simulink model "MINI_Simscape_Assignment_03"  (R2020b)
settings: Solver=FixedStepAuto  StartTime=0.0  StopTime=10  FixedStep=0.001  MaxStep=0.01  RelTol=1e-3
InitFcn:
  | parameters;
model workspace: external: MATLAB File /Users/toricolthurst/School/ECE598IntroToHumanoid/git_humanoid/Project_Matlab/Simulation_DataFile.m (data not in the file)
values from neighbouring files (symbols this model uses):
  Butter_order = 4    [parameters.m]
  Butter_order_IMU = 8    [parameters.m]
undefined symbols (not defined in the file or in its folder): smiData, X, Y, Z
libraries: sm_lib x382, nesl_utility x115, dsparch4 x19, simulink x1
(part 1 of 8)
settings Model: Creator=kggim2  LastModifiedBy=toricolthurst
settings ExplorerConfigSet: InternalSimMechanicsExplorerSettings="<ExplorerConfiguration><canonicalview>default</canonicalview><AnimationSetting><BasePlaybackSpeed>1.0</BasePlaybackSpeed><PlaybackSpeedFactor>1.0</PlaybackSpeedFactor></AnimationSetting><TilePanel><TileInfo><Tiles Columns=\"1\" Count=\"1\" Rows=\"1\"><Column Weight=\"1\"/><Row Weight=\"1\"/><Tile Height=\"1\" Width=\"1\" X=\"0\" Y=\"0\"/></Tiles></TileInfo><SceneInfo><SceneViewer><BGColor><R>0.800000011920928955</R><G>1</G><B>1</B></BGColor><Camera><DoPerspective>off</DoPerspective><Position><X>108.935689512798632</X><Y>53.7617455070637718</Y><Z>50.6647866990595901</Z></Position><Center><X>0.674444181912173146</X><Y>0.341777914819902773</Y><Z>0.208581845546273847</Z></Center><Up><X>-0.338601749819323006</X><Y>-0.185140442280279371</Y><Z>0.922535566605187762</Z></Up><ViewLimDist>1</ViewLimDist><YLim>0.289357950952195409</YLim><XLim>0.308353002437022183</XLim></Camera></SceneViewer></SceneInfo></TilePanel><MechEditorPanel><Cameras/><GfxPanelCameraMap/><VideoCreator><PlaybackSpeedRatio>1.0</PlaybackSpeedRatio><FrameRate>30</FrameRate><VideoFormat>MPEG-4</VideoFormat><FrameSize>auto</FrameSize></VideoCreator></MechEditorPanel></ExplorerConfiguration>"

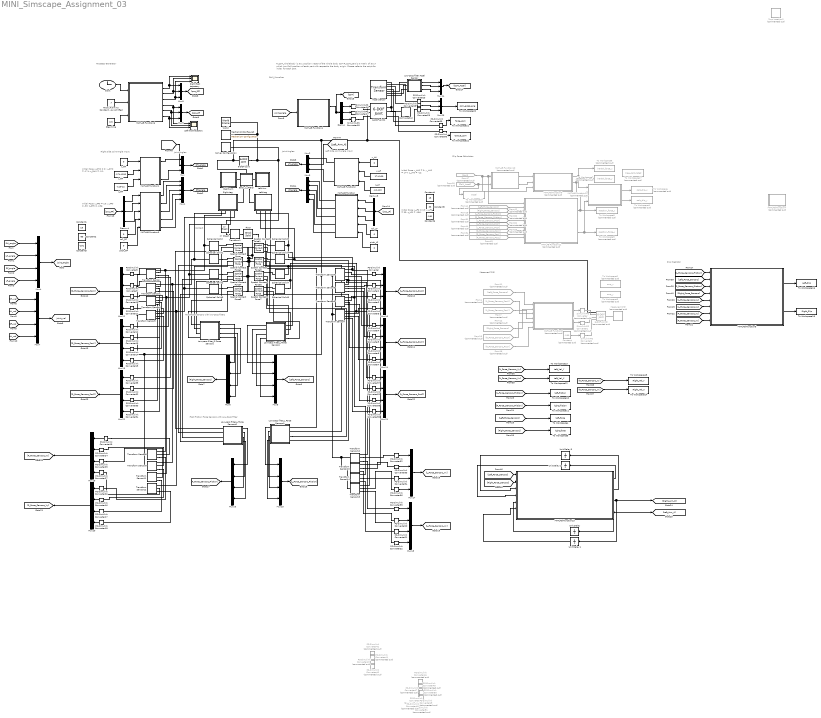
== system MINI_Simscape_Assignment_03 ==
  note: Slip Predictor
  note: P_CoM_wholebody is 3x1 position vector of the whole body CoM
      | P_CoM_part is a matrix of 3x17 which is a CoM position of each part with respect to the body origin. Please refer to the script for index for each part.
  note: Foot Force sensors with low-pass filters
  note: Footstep Generator
  note: CoM_Visualize
  note: Joint Angles
  note: Right Side Joint Angle Input
  note: Left Side Joint Angle Input
  note: Contact
  note: Joint Angles
  note: Initial Pose
      | x_RH0 = 0;
      | y_RH0 = -174;
      | z_RH0 = -12;
  note: Initial Pose
      | x_RF0 = 15;
      | y_RF0 = -33;
      | z_RF0 = -196;
  note: Initial Pose
      | x_LF0 = 15;
      | y_LF0 = 33;
      | z_LF0 = -196;
  note: Initial Pose
      | x_LH0 = 0;
      | y_LH0 = 174;
      | z_LH0 = -12;
  note: Measured ZMP
  note: Slip Force Calculator
  note: Foot Friction Force Sensors with Low-Pass Filter
  6-DOF Joint : sm_lib/Joints/6-DOF Joint  JointMode=Normal  SenseConstraintForce=off  SenseConstraintForceX=off  SenseConstraintForceY=off  SenseConstraintForceZ=off  SenseConstraintTorque=off  SenseConstraintTorqueX=off  SenseConstraintTorqueY=off  SenseConstraintTorqueZ=off  SenseTotalForce=off  SenseTotalForceX=off  SenseTotalForceY=off  SenseTotalForceZ=off  SenseTotalTorque=off  SenseTotalTorqueX=off  SenseTotalTorqueY=off  SenseTotalTorqueZ=off  CompositeWrenchDir=FollowerOnBase  CompositeWrenchFrame=BaseFrame  PxEquilibriumPosition=0  PxEquilibriumPositionUnits=m  PxSpringStiffness=0  PxSpringStiffnessUnits=N/m  PxDampingCoefficient=0  PxDampingCoefficientUnits=N/(m/s)  PxTorqueActuationMode=NoTorque  PxMotionActuationMode=ComputedMotion  PxSensePosition=off  PxSenseVelocity=off  PxSenseAcceleration=off  PxSenseTorqueForce=off  PxSenseLowerLimitTorqueForce=off  PxSenseUpperLimitTorqueForce=off  PxLowerLimitSpecify=off  PxLowerLimitBound=-1  PxLowerLimitBoundUnits=m  PxLowerLimitStiffness=1e6  PxLowerLimitStiffnessUnits=N/m  PxLowerLimitDamping=1e3  PxLowerLimitDampingUnits=N/(m/s)  PxLowerLimitTransitionRegionWidth=1e-4  PxLowerLimitTransitionRegionWidthUnits=m  PxUpperLimitSpecify=off  PxUpperLimitBound=1  PxUpperLimitBoundUnits=m  PxUpperLimitStiffness=1e6  PxUpperLimitStiffnessUnits=N/m  PxUpperLimitDamping=1e3  PxUpperLimitDampingUnits=N/(m/s)  PxUpperLimitTransitionRegionWidth=1e-4  PxUpperLimitTransitionRegionWidthUnits=m  PxPositionTargetSpecify=off  PxPositionTargetPriority=High  PxPositionTargetValue=0  PxPositionTargetValueUnits=m  PxVelocityTargetSpecify=off  PxVelocityTargetPriority=High  PxVelocityTargetValue=0  PxVelocityTargetValueUnits=m/s  PyEquilibriumPosition=0  PyEquilibriumPositionUnits=m  PySpringStiffness=0  PySpringStiffnessUnits=N/m  PyDampingCoefficient=0  PyDampingCoefficientUnits=N/(m/s)  PyTorqueActuationMode=NoTorque  PyMotionActuationMode=ComputedMotion  PySensePosition=off  PySenseVelocity=off  PySenseAcceleration=off  PySenseTorqueForce=off  PySenseLowerLimitTorqueForce=off  PySenseUpperLimitTorqueForce=off  PyLowerLimitSpecify=off  PyLowerLimitBound=-1  PyLowerLimitBoundUnits=m  PyLowerLimitStiffness=1e6  PyLowerLimitStiffnessUnits=N/m  PyLowerLimitDamping=1e3  PyLowerLimitDampingUnits=N/(m/s)  PyLowerLimitTransitionRegionWidth=1e-4  PyLowerLimitTransitionRegionWidthUnits=m  PyUpperLimitSpecify=off  PyUpperLimitBound=1  PyUpperLimitBoundUnits=m  PyUpperLimitStiffness=1e6  PyUpperLimitStiffnessUnits=N/m  PyUpperLimitDamping=1e3  PyUpperLimitDampingUnits=N/(m/s)  PyUpperLimitTransitionRegionWidth=1e-4  PyUpperLimitTransitionRegionWidthUnits=m  PyPositionTargetSpecify=off  PyPositionTargetPriority=High  PyPositionTargetValue=0  PyPositionTargetValueUnits=m  PyVelocityTargetSpecify=off  PyVelocityTargetPriority=High  PyVelocityTargetValue=0  PyVelocityTargetValueUnits=m/s  PzEquilibriumPosition=0  PzEquilibriumPositionUnits=m  PzSpringStiffness=0  PzSpringStiffnessUnits=N/m  PzDampingCoefficient=0  PzDampingCoefficientUnits=N/(m/s)  PzTorqueActuationMode=NoTorque  PzMotionActuationMode=ComputedMotion  PzSensePosition=off  PzSenseVelocity=off  PzSenseAcceleration=off  PzSenseTorqueForce=off  PzSenseLowerLimitTorqueForce=off  PzSenseUpperLimitTorqueForce=off  PzLowerLimitSpecify=off  PzLowerLimitBound=-1  PzLowerLimitBoundUnits=m  PzLowerLimitStiffness=1e6  PzLowerLimitStiffnessUnits=N/m  PzLowerLimitDamping=1e3  PzLowerLimitDampingUnits=N/(m/s)  PzLowerLimitTransitionRegionWidth=1e-4  PzLowerLimitTransitionRegionWidthUnits=m  PzUpperLimitSpecify=off  PzUpperLimitBound=1  PzUpperLimitBoundUnits=m  PzUpperLimitStiffness=1e6  PzUpperLimitStiffnessUnits=N/m  PzUpperLimitDamping=1e3  PzUpperLimitDampingUnits=N/(m/s)  PzUpperLimitTransitionRegionWidth=1e-4  PzUpperLimitTransitionRegionWidthUnits=m  PzPositionTargetSpecify=off  PzPositionTargetPriority=High  PzPositionTargetValue=0  PzPositionTargetValueUnits=m  PzVelocityTargetSpecify=off  PzVelocityTargetPriority=High  PzVelocityTargetValue=0  PzVelocityTargetValueUnits=m/s  SphDefPosRotationMethod=None  SphDefPosRotationAngleUnits=deg  SphDefPosRotationStandardAxis=+Z  SphDefPosRotationAngle=0.0  SphDefPosRotationArbitraryAxis=[0 0 1]  SphDefPosFollAlignAxisA=+X  SphDefPosBaseAlignAxisA=+Y  SphDefPosFollAlignAxisB=+Y  SphDefPosBaseAlignAxisB=+Z  SphDefPosRotationSequenceAxes=FollowerAxes  SphDefPosRotationSequence=XYX  SphDefPosRotationSequenceAngles=[0 0 0]  SphDefPosRotationSequenceAnglesUnits=deg  SphDefPosRotationMatrix=[1 0 0; 0 1 0; 0 0 1]  SphEqPosRotationMethod=None  SphEqPosRotationAngleUnits=deg  SphEqPosRotationStandardAxis=+Z  SphEqPosRotationAngle=0.0  SphEqPosRotationArbitraryAxis=[0 0 1]  SphEqPosFollAlignAxisA=+X  SphEqPosBaseAlignAxisA=+Y  SphEqPosFollAlignAxisB=+Y  SphEqPosBaseAlignAxisB=+Z  SphEqPosRotationSequenceAxes=FollowerAxes  SphEqPosRotationSequence=XYX  SphEqPosRotationSequenceAngles=[0 0 0]  SphEqPosRotationSequenceAnglesUnits=deg  SphEqPosRotationMatrix=[1 0 0; 0 1 0; 0 0 1]  SphSpringStiffness=0  SphSpringStiffnessUnits=N*m/deg  SphDampingCoefficient=0  SphDampingCoefficientUnits=N*m/(deg/s)  SphActuateTorqueX=off  SphActuateTorqueY=off  SphActuateTorqueZ=off  SphActuateTorque=off  SphTorqueActuationMode=NoTorque  SphMotionActuationMode=ComputedMotion  SphActuationFrame=BaseFrame  SphSensePosition=off  SphSenseVelocityX=off  SphSenseVelocityY=off  SphSenseVelocityZ=off  SphSenseVelocity=off  SphSenseAccelerationX=off  SphSenseAccelerationY=off  SphSenseAccelerationZ=off  SphSenseAcceleration=off  SphSenseTorqueX=off  SphSenseTorqueY=off  SphSenseTorqueZ=off  SphSenseTorqueForce=off  SphSenseLowerLimitTorqueMag=off  SphSenseUpperLimitTorqueMag=off  SphSensingFrame=BaseFrame  SphLowerLimitSpecify=off  SphLowerLimitBound=15  SphLowerLimitBoundUnits=deg  SphLowerLimitStiffness=1e4  SphLowerLimitStiffnessUnits=N*m/deg  SphLowerLimitDamping=10  SphLowerLimitDampingUnits=N*m/(deg/s)  SphLowerLimitTransitionRegionWidth=0.1  SphLowerLimitTransitionRegionWidthUnits=deg  SphUpperLimitSpecify=off  SphUpperLimitBound=45  SphUpperLimitBoundUnits=deg  SphUpperLimitStiffness=1e4  SphUpperLimitStiffnessUnits=N*m/deg  SphUpperLimitDamping=10  SphUpperLimitDampingUnits=N*m/(deg/s)  SphUpperLimitTransitionRegionWidth=0.1  SphUpperLimitTransitionRegionWidthUnits=deg  SphPositionTargetRotationMethod=None  SphPositionTargetRotationAngleUnits=deg  SphPositionTargetRotationStandardAxis=+Z  SphPositionTargetRotationAngle=0.0  SphPositionTargetRotationArbitraryAxis=[0 0 1]  SphPositionTargetFollAlignAxisA=+X  SphPositionTargetBaseAlignAxisA=+Y  SphPositionTargetFollAlignAxisB=+Y  SphPositionTargetBaseAlignAxisB=+Z  SphPositionTargetRotationSequenceAxes=FollowerAxes  SphPositionTargetRotationSequence=XYX  SphPositionTargetRotationSequenceAngles=[0 0 0]  SphPositionTargetRotationSequenceAnglesUnits=deg  SphPositionTargetRotationMatrix=[1 0 0; 0 1 0; 0 0 1]  SphPositionTargetSpecify=off  SphPositionTargetPriority=High  SphVelocityTargetValue=[0 0 0]  SphVelocityTargetValueUnits=deg/s  SphVelocityTargetSpecify=off  SphVelocityTargetPriority=High  SphVelocityTargetInFollowerFrame=on
  6-DOF Joint1 : sm_lib/Joints/6-DOF Joint  JointMode=Normal  SenseConstraintForce=off  SenseConstraintForceX=off  SenseConstraintForceY=off  SenseConstraintForceZ=off  SenseConstraintTorque=off  SenseConstraintTorqueX=off  SenseConstraintTorqueY=off  SenseConstraintTorqueZ=off  SenseTotalForce=on  SenseTotalForceX=off  SenseTotalForceY=off  SenseTotalForceZ=off  SenseTotalTorque=on  SenseTotalTorqueX=off  SenseTotalTorqueY=off  SenseTotalTorqueZ=off  CompositeWrenchDir=FollowerOnBase  CompositeWrenchFrame=BaseFrame  PxEquilibriumPosition=0  PxEquilibriumPositionUnits=m  PxSpringStiffness=0  PxSpringStiffnessUnits=N/m  PxDampingCoefficient=0  PxDampingCoefficientUnits=N/(m/s)  PxTorqueActuationMode=ComputedTorque  PxMotionActuationMode=InputMotion  PxSensePosition=off  PxSenseVelocity=off  PxSenseAcceleration=off  PxSenseTorqueForce=off  PxSenseLowerLimitTorqueForce=off  PxSenseUpperLimitTorqueForce=off  PxLowerLimitSpecify=off  PxLowerLimitBound=-1  PxLowerLimitBoundUnits=m  PxLowerLimitStiffness=1e6  PxLowerLimitStiffnessUnits=N/m  PxLowerLimitDamping=1e3  PxLowerLimitDampingUnits=N/(m/s)  PxLowerLimitTransitionRegionWidth=1e-4  PxLowerLimitTransitionRegionWidthUnits=m  PxUpperLimitSpecify=off  PxUpperLimitBound=1  PxUpperLimitBoundUnits=m  PxUpperLimitStiffness=1e6  PxUpperLimitStiffnessUnits=N/m  PxUpperLimitDamping=1e3  PxUpperLimitDampingUnits=N/(m/s)  PxUpperLimitTransitionRegionWidth=1e-4  PxUpperLimitTransitionRegionWidthUnits=m  PxPositionTargetSpecify=off  PxPositionTargetPriority=High  PxPositionTargetValue=0  PxPositionTargetValueUnits=m  PxVelocityTargetSpecify=off  PxVelocityTargetPriority=High  PxVelocityTargetValue=0  PxVelocityTargetValueUnits=m/s  PyEquilibriumPosition=0  PyEquilibriumPositionUnits=m  PySpringStiffness=0  PySpringStiffnessUnits=N/m  PyDampingCoefficient=0  PyDampingCoefficientUnits=N/(m/s)  PyTorqueActuationMode=ComputedTorque  PyMotionActuationMode=InputMotion  PySensePosition=off  PySenseVelocity=off  PySenseAcceleration=off  PySenseTorqueForce=off  PySenseLowerLimitTorqueForce=off  PySenseUpperLimitTorqueForce=off  PyLowerLimitSpecify=off  PyLowerLimitBound=-1  PyLowerLimitBoundUnits=m  PyLowerLimitStiffness=1e6  PyLowerLimitStiffnessUnits=N/m  PyLowerLimitDamping=1e3  PyLowerLimitDampingUnits=N/(m/s)  PyLowerLimitTransitionRegionWidth=1e-4  PyLowerLimitTransitionRegionWidthUnits=m  PyUpperLimitSpecify=off  PyUpperLimitBound=1  PyUpperLimitBoundUnits=m  PyUpperLimitStiffness=1e6  PyUpperLimitStiffnessUnits=N/m  PyUpperLimitDamping=1e3  PyUpperLimitDampingUnits=N/(m/s)  PyUpperLimitTransitionRegionWidth=1e-4  PyUpperLimitTransitionRegionWidthUnits=m  PyPositionTargetSpecify=off  PyPositionTargetPriority=High  PyPositionTargetValue=0  PyPositionTargetValueUnits=m  PyVelocityTargetSpecify=off  PyVelocityTargetPriority=High  PyVelocityTargetValue=0  PyVelocityTargetValueUnits=m/s  PzEquilibriumPosition=0  PzEquilibriumPositionUnits=m  PzSpringStiffness=0  PzSpringStiffnessUnits=N/m  PzDampingCoefficient=0  PzDampingCoefficientUnits=N/(m/s)  PzTorqueActuationMode=ComputedTorque  PzMotionActuationMode=InputMotion  PzSensePosition=off  PzSenseVelocity=off  PzSenseAcceleration=off  PzSenseTorqueForce=off  PzSenseLowerLimitTorqueForce=off  PzSenseUpperLimitTorqueForce=off  PzLowerLimitSpecify=off  PzLowerLimitBound=-1  PzLowerLimitBoundUnits=m  PzLowerLimitStiffness=1e6  PzLowerLimitStiffnessUnits=N/m  PzLowerLimitDamping=1e3  PzLowerLimitDampingUnits=N/(m/s)  PzLowerLimitTransitionRegionWidth=1e-4  PzLowerLimitTransitionRegionWidthUnits=m  PzUpperLimitSpecify=off  PzUpperLimitBound=1  PzUpperLimitBoundUnits=m  PzUpperLimitStiffness=1e6  PzUpperLimitStiffnessUnits=N/m  PzUpperLimitDamping=1e3  PzUpperLimitDampingUnits=N/(m/s)  PzUpperLimitTransitionRegionWidth=1e-4  PzUpperLimitTransitionRegionWidthUnits=m  PzPositionTargetSpecify=off  PzPositionTargetPriority=High  PzPositionTargetValue=0  PzPositionTargetValueUnits=m  PzVelocityTargetSpecify=off  PzVelocityTargetPriority=High  PzVelocityTargetValue=0  PzVelocityTargetValueUnits=m/s  SphDefPosRotationMethod=None  SphDefPosRotationAngleUnits=deg  SphDefPosRotationStandardAxis=+Z  SphDefPosRotationAngle=0.0  SphDefPosRotationArbitraryAxis=[0 0 1]  SphDefPosFollAlignAxisA=+X  SphDefPosBaseAlignAxisA=+Y  SphDefPosFollAlignAxisB=+Y  SphDefPosBaseAlignAxisB=+Z  SphDefPosRotationSequenceAxes=FollowerAxes  SphDefPosRotationSequence=XYX  SphDefPosRotationSequenceAngles=[0 0 0]  SphDefPosRotationSequenceAnglesUnits=deg  SphDefPosRotationMatrix=[1 0 0; 0 1 0; 0 0 1]  SphEqPosRotationMethod=None  SphEqPosRotationAngleUnits=deg  SphEqPosRotationStandardAxis=+Z  SphEqPosRotationAngle=0.0  SphEqPosRotationArbitraryAxis=[0 0 1]  SphEqPosFollAlignAxisA=+X  SphEqPosBaseAlignAxisA=+Y  SphEqPosFollAlignAxisB=+Y  SphEqPosBaseAlignAxisB=+Z  SphEqPosRotationSequenceAxes=FollowerAxes  SphEqPosRotationSequence=XYX  SphEqPosRotationSequenceAngles=[0 0 0]  SphEqPosRotationSequenceAnglesUnits=deg  SphEqPosRotationMatrix=[1 0 0; 0 1 0; 0 0 1]  SphSpringStiffness=0  SphSpringStiffnessUnits=N*m/deg  SphDampingCoefficient=0  SphDampingCoefficientUnits=N*m/(deg/s)  SphActuateTorqueX=off  SphActuateTorqueY=off  SphActuateTorqueZ=off  SphActuateTorque=off  SphTorqueActuationMode=NoTorque  SphMotionActuationMode=ComputedMotion  SphActuationFrame=BaseFrame  SphSensePosition=off  SphSenseVelocityX=off  SphSenseVelocityY=off  SphSenseVelocityZ=off  SphSenseVelocity=off  SphSenseAccelerationX=off  SphSenseAccelerationY=off  SphSenseAccelerationZ=off  SphSenseAcceleration=off  SphSenseTorqueX=off  SphSenseTorqueY=off  SphSenseTorqueZ=off  SphSenseTorqueForce=off  SphSenseLowerLimitTorqueMag=off  SphSenseUpperLimitTorqueMag=off  SphSensingFrame=BaseFrame  SphLowerLimitSpecify=off  SphLowerLimitBound=15  SphLowerLimitBoundUnits=deg  SphLowerLimitStiffness=1e4  SphLowerLimitStiffnessUnits=N*m/deg  SphLowerLimitDamping=10  SphLowerLimitDampingUnits=N*m/(deg/s)  SphLowerLimitTransitionRegionWidth=0.1  SphLowerLimitTransitionRegionWidthUnits=deg  SphUpperLimitSpecify=off  SphUpperLimitBound=45  SphUpperLimitBoundUnits=deg  SphUpperLimitStiffness=1e4  SphUpperLimitStiffnessUnits=N*m/deg  SphUpperLimitDamping=10  SphUpperLimitDampingUnits=N*m/(deg/s)  SphUpperLimitTransitionRegionWidth=0.1  SphUpperLimitTransitionRegionWidthUnits=deg  SphPositionTargetRotationMethod=None  SphPositionTargetRotationAngleUnits=deg  SphPositionTargetRotationStandardAxis=+Z  SphPositionTargetRotationAngle=0.0  SphPositionTargetRotationArbitraryAxis=[0 0 1]  SphPositionTargetFollAlignAxisA=+X  SphPositionTargetBaseAlignAxisA=+Y  SphPositionTargetFollAlignAxisB=+Y  SphPositionTargetBaseAlignAxisB=+Z  SphPositionTargetRotationSequenceAxes=FollowerAxes  SphPositionTargetRotationSequence=XYX  SphPositionTargetRotationSequenceAngles=[0 0 0]  SphPositionTargetRotationSequenceAnglesUnits=deg  SphPositionTargetRotationMatrix=[1 0 0; 0 1 0; 0 0 1]  SphPositionTargetSpecify=off  SphPositionTargetPriority=High  SphVelocityTargetValue=[0 0 0]  SphVelocityTargetValueUnits=deg/s  SphVelocityTargetSpecify=off  SphVelocityTargetPriority=High  SphVelocityTargetInFollowerFrame=on
  6-DOF Joint2 : sm_lib/Joints/6-DOF Joint  Commented=on  JointMode=Normal  SenseConstraintForce=off  SenseConstraintForceX=off  SenseConstraintForceY=off  SenseConstraintForceZ=off  SenseConstraintTorque=off  SenseConstraintTorqueX=off  SenseConstraintTorqueY=off  SenseConstraintTorqueZ=off  SenseTotalForce=off  SenseTotalForceX=off  SenseTotalForceY=off  SenseTotalForceZ=off  SenseTotalTorque=off  SenseTotalTorqueX=off  SenseTotalTorqueY=off  SenseTotalTorqueZ=off  CompositeWrenchDir=FollowerOnBase  CompositeWrenchFrame=BaseFrame  PxEquilibriumPosition=0  PxEquilibriumPositionUnits=m  PxSpringStiffness=0  PxSpringStiffnessUnits=N/m  PxDampingCoefficient=0  PxDampingCoefficientUnits=N/(m/s)  PxTorqueActuationMode=ComputedTorque  PxMotionActuationMode=InputMotion  PxSensePosition=off  PxSenseVelocity=off  PxSenseAcceleration=off  PxSenseTorqueForce=off  PxSenseLowerLimitTorqueForce=off  PxSenseUpperLimitTorqueForce=off  PxLowerLimitSpecify=off  PxLowerLimitBound=-1  PxLowerLimitBoundUnits=m  PxLowerLimitStiffness=1e6  PxLowerLimitStiffnessUnits=N/m  PxLowerLimitDamping=1e3  PxLowerLimitDampingUnits=N/(m/s)  PxLowerLimitTransitionRegionWidth=1e-4  PxLowerLimitTransitionRegionWidthUnits=m  PxUpperLimitSpecify=off  PxUpperLimitBound=1  PxUpperLimitBoundUnits=m  PxUpperLimitStiffness=1e6  PxUpperLimitStiffnessUnits=N/m  PxUpperLimitDamping=1e3  PxUpperLimitDampingUnits=N/(m/s)  PxUpperLimitTransitionRegionWidth=1e-4  PxUpperLimitTransitionRegionWidthUnits=m  PxPositionTargetSpecify=off  PxPositionTargetPriority=High  PxPositionTargetValue=0  PxPositionTargetValueUnits=m  PxVelocityTargetSpecify=off  PxVelocityTargetPriority=High  PxVelocityTargetValue=0  PxVelocityTargetValueUnits=m/s  PyEquilibriumPosition=0  PyEquilibriumPositionUnits=m  PySpringStiffness=0  PySpringStiffnessUnits=N/m  PyDampingCoefficient=0  PyDampingCoefficientUnits=N/(m/s)  PyTorqueActuationMode=ComputedTorque  PyMotionActuationMode=InputMotion  PySensePosition=off  PySenseVelocity=off  PySenseAcceleration=off  PySenseTorqueForce=off  PySenseLowerLimitTorqueForce=off  PySenseUpperLimitTorqueForce=off  PyLowerLimitSpecify=off  PyLowerLimitBound=-1  PyLowerLimitBoundUnits=m  PyLowerLimitStiffness=1e6  PyLowerLimitStiffnessUnits=N/m  PyLowerLimitDamping=1e3  PyLowerLimitDampingUnits=N/(m/s)  PyLowerLimitTransitionRegionWidth=1e-4  PyLowerLimitTransitionRegionWidthUnits=m  PyUpperLimitSpecify=off  PyUpperLimitBound=1  PyUpperLimitBoundUnits=m  PyUpperLimitStiffness=1e6  PyUpperLimitStiffnessUnits=N/m  PyUpperLimitDamping=1e3  PyUpperLimitDampingUnits=N/(m/s)  PyUpperLimitTransitionRegionWidth=1e-4  PyUpperLimitTransitionRegionWidthUnits=m  PyPositionTargetSpecify=off  PyPositionTargetPriority=High  PyPositionTargetValue=0  PyPositionTargetValueUnits=m  PyVelocityTargetSpecify=off  PyVelocityTargetPriority=High  PyVelocityTargetValue=0  PyVelocityTargetValueUnits=m/s  PzEquilibriumPosition=0  PzEquilibriumPositionUnits=m  PzSpringStiffness=0  PzSpringStiffnessUnits=N/m  PzDampingCoefficient=0  PzDampingCoefficientUnits=N/(m/s)  PzTorqueActuationMode=ComputedTorque  PzMotionActuationMode=InputMotion  PzSensePosition=off  PzSenseVelocity=off  PzSenseAcceleration=off  PzSenseTorqueForce=off  PzSenseLowerLimitTorqueForce=off  PzSenseUpperLimitTorqueForce=off  PzLowerLimitSpecify=off  PzLowerLimitBound=-1  PzLowerLimitBoundUnits=m  PzLowerLimitStiffness=1e6  PzLowerLimitStiffnessUnits=N/m  PzLowerLimitDamping=1e3  PzLowerLimitDampingUnits=N/(m/s)  PzLowerLimitTransitionRegionWidth=1e-4  PzLowerLimitTransitionRegionWidthUnits=m  PzUpperLimitSpecify=off  PzUpperLimitBound=1  PzUpperLimitBoundUnits=m  PzUpperLimitStiffness=1e6  PzUpperLimitStiffnessUnits=N/m  PzUpperLimitDamping=1e3  PzUpperLimitDampingUnits=N/(m/s)  PzUpperLimitTransitionRegionWidth=1e-4  PzUpperLimitTransitionRegionWidthUnits=m  PzPositionTargetSpecify=off  PzPositionTargetPriority=High  PzPositionTargetValue=0  PzPositionTargetValueUnits=m  PzVelocityTargetSpecify=off  PzVelocityTargetPriority=High  PzVelocityTargetValue=0  PzVelocityTargetValueUnits=m/s  SphDefPosRotationMethod=None  SphDefPosRotationAngleUnits=deg  SphDefPosRotationStandardAxis=+Z  SphDefPosRotationAngle=0.0  SphDefPosRotationArbitraryAxis=[0 0 1]  SphDefPosFollAlignAxisA=+X  SphDefPosBaseAlignAxisA=+Y  SphDefPosFollAlignAxisB=+Y  SphDefPosBaseAlignAxisB=+Z  SphDefPosRotationSequenceAxes=FollowerAxes  SphDefPosRotationSequence=XYX  SphDefPosRotationSequenceAngles=[0 0 0]  SphDefPosRotationSequenceAnglesUnits=deg  SphDefPosRotationMatrix=[1 0 0; 0 1 0; 0 0 1]  SphEqPosRotationMethod=None  SphEqPosRotationAngleUnits=deg  SphEqPosRotationStandardAxis=+Z  SphEqPosRotationAngle=0.0  SphEqPosRotationArbitraryAxis=[0 0 1]  SphEqPosFollAlignAxisA=+X  SphEqPosBaseAlignAxisA=+Y  SphEqPosFollAlignAxisB=+Y  SphEqPosBaseAlignAxisB=+Z  SphEqPosRotationSequenceAxes=FollowerAxes  SphEqPosRotationSequence=XYX  SphEqPosRotationSequenceAngles=[0 0 0]  SphEqPosRotationSequenceAnglesUnits=deg  SphEqPosRotationMatrix=[1 0 0; 0 1 0; 0 0 1]  SphSpringStiffness=0  SphSpringStiffnessUnits=N*m/deg  SphDampingCoefficient=0  SphDampingCoefficientUnits=N*m/(deg/s)  SphActuateTorqueX=off  SphActuateTorqueY=off  SphActuateTorqueZ=off  SphActuateTorque=off  SphTorqueActuationMode=NoTorque  SphMotionActuationMode=ComputedMotion  SphActuationFrame=BaseFrame  SphSensePosition=off  SphSenseVelocityX=off  SphSenseVelocityY=off  SphSenseVelocityZ=off  SphSenseVelocity=off  SphSenseAccelerationX=off  SphSenseAccelerationY=off  SphSenseAccelerationZ=off  SphSenseAcceleration=off  SphSenseTorqueX=off  SphSenseTorqueY=off  SphSenseTorqueZ=off  SphSenseTorqueForce=off  SphSenseLowerLimitTorqueMag=off  SphSenseUpperLimitTorqueMag=off  SphSensingFrame=BaseFrame  SphLowerLimitSpecify=off  SphLowerLimitBound=15  SphLowerLimitBoundUnits=deg  SphLowerLimitStiffness=1e4  SphLowerLimitStiffnessUnits=N*m/deg  SphLowerLimitDamping=10  SphLowerLimitDampingUnits=N*m/(deg/s)  SphLowerLimitTransitionRegionWidth=0.1  SphLowerLimitTransitionRegionWidthUnits=deg  SphUpperLimitSpecify=off  SphUpperLimitBound=45  SphUpperLimitBoundUnits=deg  SphUpperLimitStiffness=1e4  SphUpperLimitStiffnessUnits=N*m/deg  SphUpperLimitDamping=10  SphUpperLimitDampingUnits=N*m/(deg/s)  SphUpperLimitTransitionRegionWidth=0.1  SphUpperLimitTransitionRegionWidthUnits=deg  SphPositionTargetRotationMethod=None  SphPositionTargetRotationAngleUnits=deg  SphPositionTargetRotationStandardAxis=+Z  SphPositionTargetRotationAngle=0.0  SphPositionTargetRotationArbitraryAxis=[0 0 1]  SphPositionTargetFollAlignAxisA=+X  SphPositionTargetBaseAlignAxisA=+Y  SphPositionTargetFollAlignAxisB=+Y  SphPositionTargetBaseAlignAxisB=+Z  SphPositionTargetRotationSequenceAxes=FollowerAxes  SphPositionTargetRotationSequence=XYX  SphPositionTargetRotationSequenceAngles=[0 0 0]  SphPositionTargetRotationSequenceAnglesUnits=deg  SphPositionTargetRotationMatrix=[1 0 0; 0 1 0; 0 0 1]  SphPositionTargetSpecify=off  SphPositionTargetPriority=High  SphVelocityTargetValue=[0 0 0]  SphVelocityTargetValueUnits=deg/s  SphVelocityTargetSpecify=off  SphVelocityTargetPriority=High  SphVelocityTargetInFollowerFrame=on
  Accel Sensor : sm_lib/Frames and Transforms/Transform Sensor  MeasurementFrame=World  SenseAngle=off  SenseAxis=off  SenseAngle1=off  SenseAngle2=off  SenseAngle3=off  SenseQ=off  SenseR=off  SenseOmegaX=off  SenseOmegaY=off  SenseOmegaZ=off  SenseOmega1=off  SenseOmega2=off  SenseOmega3=off  SenseQDot=off  SenseRDot=off  SenseAlphaX=on  SenseAlphaY=on  SenseAlphaZ=on  SenseAlpha1=off  SenseAlpha2=off  SenseAlpha3=off  SenseQDDot=off  SenseRDDot=off  SenseX=off  SenseY=off  SenseZ=off  SenseRad=off  SenseAzim=off  SenseDist=off  SenseInc=off  SenseXDot=off  SenseYDot=off  SenseZDot=off  SenseRadDot=off  SenseAzimDot=off  SenseDistDot=off  SenseIncDot=off  SenseXDDot=on  SenseYDDot=on  SenseZDDot=on  SenseRadDDot=off  SenseAzimDDot=off  SenseDistDDot=off  SenseIncDDot=off
  Body_1_RIGID : Subsystem
      settings: PortSchema="{\"entries\":[{\"content\":{\"sides\":[{\"content\":{\"connectorIds\":[\"LConn1\"]},\"type\":\"ConnectorPlacement.EquallySpacedRectSide\",\"uuid\":\"75841b4a-1b72-41b2-8013-c129c8e49b08\"},{\"content\":{\"connectorIds\":[\"RConn1\"],\"side\":\"RIGHT\"},\"type\":\"ConnectorPlacement.EquallySpacedRectSide\",\"uuid\":\"41ac541f-18a4-47e5-a096-fba9b85426fc\"},{\"content\":{\"connectorIds\":[\"LConn2\"],\"side\":\"TOP\"},\"type\":\"ConnectorPlacement.EquallySpacedRectSide\",\"uuid\":\"13cc0822-4502-483f-b652-853a4ab24169\"},{\"content\":{\"connectorIds\":[\"RConn2\",\"RConn3\"],\"side\":\"BOTTOM\"},\"type\":\"ConnectorPlacement.EquallySpacedRectSide\",\"uuid\":\"f29663d4-322e-486e-a81b-251c763aaf27\"}]},\"type\":\"ConnectorPlacement.EquallySpacedConnector\",\"uuid\":\"7bf843b2-abd3-472f-bd55-2383dc6cc087\"}],\"packageUris\":[\"http://schema.mathworks.com/mf0/Connector/19700101\"],\"version\":\"1.0\"}"
  "Clock " : Clock
  CoM Location : sm_lib/Body Elements/Spherical Solid  GraphicAmbientColor=[0.15 0.15 0.15 1.0]  BasedOnType=Density  CenterOfMass=[0 0 0]  CenterOfMassUnits=m  GraphicDiffuseColor=CoM_color  Density=0.001  DensityUnits=kg/m^3  DoExposeReferenceFrame=on  GraphicEmissiveColor=[0.0 0.0 0.0 1.0]  ExportEntireGeometry=off  SerializedExposedGeometries=<ExposedGeometries/>  SerializedFrames=<Frames/>  MarkerShape=Sphere  MarkerSize=10  GraphicType=FromGeometry  InertiaType=CalculateFromGeometry  Mass=1  MassUnits=kg  MomentsOfInertia=[1 1 1]  MomentsOfInertiaUnits=kg*m^2  GraphicOpacity=1  ProductsOfInertia=[0 0 0]  ProductsOfInertiaUnits=kg*m^2  GraphicShininess=75  GraphicSpecularColor=[0.5 0.5 0.5 1.0]  SphereRadius=CoM_r  SphereRadiusUnits=mm  GraphicVisPropType=SimpleVisualProperties
  Constant : Constant  Commented=on  Value=-190
  Constant1 : Constant  Value=15
  Constant2 : Constant  Value=-33
  Constant3 : Constant  Value=-191
  Constant4 : Constant  Value=15
  Constant5 : Constant  Value=33
  Constant6 : Constant  Value=-191
  Demux : Demux  Outputs=3
  Demux4 : Demux  Outputs=3
  Demux5 : Demux  Outputs=3
  Floor : sm_lib/Body Elements/Brick Solid  GraphicAmbientColor=[0.15 0.15 0.15 1.0]  BasedOnType=Density  BrickDimensions=[2 2 0.005]  BrickDimensionUnits=m  CenterOfMass=[0 0 0]  CenterOfMassUnits=m  GraphicDiffuseColor=[0.0 1.0 0.2]  Density=1000  DensityUnits=kg/m^3  DoExposeReferenceFrame=on  GraphicEmissiveColor=[0.0 0.0 0.0 1.0]  ExportEntireGeometry=on  SerializedFrames=<Frames/>  MarkerShape=Sphere  MarkerSize=10  GraphicType=FromGeometry  InertiaType=CalculateFromGeometry  Mass=1  MassUnits=kg  MomentsOfInertia=[1 1 1]  MomentsOfInertiaUnits=kg*m^2  GraphicOpacity=0.3  ProductsOfInertia=[0 0 0]  ProductsOfInertiaUnits=kg*m^2  GraphicShininess=75  GraphicSpecularColor=[0.5 0.5 0.5 1.0]  GraphicVisPropType=SimpleVisualProperties
  "Foot Lift timing Constant (0~1) if 0, feet are not lifted" : Constant  Value=.7
  From11 : From  Commented=on  GotoTag=Left_Force_Sensors
  From12 : From  Commented=on  GotoTag=Right_Force_Sensors
  From15 : From  Commented=on  GotoTag=R_Force_Sensors_PosX
  From16 : From  Commented=on  GotoTag=R_Force_Sensors_PosY
  From17 : From  Commented=on  GotoTag=CoM
  From18 : From  Commented=on  GotoTag=CoM_Accel
  From29 : From  Commented=on  GotoTag=L_Force_Sensors_Friction
  From30 : From  Commented=on  GotoTag=R_Force_Sensors_Friction
  From31 : From  Commented=on  GotoTag=L_Force_Sensors_PosX
  From32 : From  Commented=on  GotoTag=L_Force_Sensors_PosY
  From33 : From  Commented=on  GotoTag=R_Force_Sensors_PosX
  From34 : From  Commented=on  GotoTag=R_Force_Sensors_PosY
  From4 : From  Commented=on  GotoTag=L_Force_Sensors_PosX
  From41 : From  Commented=on  GotoTag=Left_Force_Sensors
  From42 : From  Commented=on  GotoTag=Right_Force_Sensors
  From43 : From  Commented=on  GotoTag=R_Force_Sensors_PosZ
  From44 : From  Commented=on  GotoTag=L_Force_Sensors_PosX
  From7 : From  Commented=on  GotoTag=L_Force_Sensors_PosY
  Left Arm : Subsystem
  Left Leg : Subsystem
      settings: PortSchema="{\"entries\":[{\"content\":{\"sides\":[{\"content\":{\"connectorIds\":[]},\"type\":\"ConnectorPlacement.EquallySpacedRectSide\",\"uuid\":\"9e969ea6-e951-4d4a-bf57-ef557d09f6a3\"},{\"content\":{\"connectorIds\":[\"RConn1\",\"RConn2\",\"RConn3\",\"RConn4\"],\"side\":\"RIGHT\"},\"type\":\"ConnectorPlacement.EquallySpacedRectSide\",\"uuid\":\"8f3efddf-64bc-4e54-80b2-49157da9b6a5\"},{\"content\":{\"connectorIds\":[\"LConn1\"],\"side\":\"TOP\"},\"type\":\"ConnectorPlacement.EquallySpacedRectSide\",\"uuid\":\"165993f7-6b81-43bd-a5ce-b1e99e25c667\"},{\"content\":{\"connectorIds\":[],\"side\":\"HIDDEN\"},\"type\":\"ConnectorPlacement.EquallySpacedRectSide\",\"uuid\":\"8667408d-6e34-4966-9d08-787d76b6f64b\"}]},\"type\":\"ConnectorPlacement.EquallySpacedConnector\",\"uuid\":\"f5cb6cb1-f1fe-4377-a43e-e6f81aaebafd\"}],\"packageUris\":[\"http://schema.mathworks.com/mf0/Connector/R2020b\"],\"version\":\"1.0\"}"
  Left foot trajectory : Scope  NumInputPorts=3
  Low-pass filter Accel Sensor : Subsystem
  Low-pass filter_L Force Sensors : Subsystem
  Low-pass filter_L Force Sensors1 : Subsystem
  Low-pass filter_L Force Sensors2 : Subsystem
  Low-pass filter_R Force Sensors : Subsystem
  MATLAB Function : MATLAB Function  TreatAsAtomicUnit=on
  MATLAB Function1 : MATLAB Function  TreatAsAtomicUnit=on
  MATLAB Function10 : MATLAB Function  Commented=on  TreatAsAtomicUnit=on
  MATLAB Function11 : MATLAB Function  Commented=on  TreatAsAtomicUnit=on
  MATLAB Function12 : MATLAB Function  Commented=on  TreatAsAtomicUnit=on
  MATLAB Function13 : MATLAB Function  TreatAsAtomicUnit=on
  MATLAB Function2 : MATLAB Function  TreatAsAtomicUnit=on
  MATLAB Function3 : MATLAB Function  TreatAsAtomicUnit=on
  MATLAB Function4 : MATLAB Function  ClipboardFcn=DHparameter; RX; RY; RZ; TXYZ;  TreatAsAtomicUnit=on
  MATLAB Function5 : MATLAB Function  TreatAsAtomicUnit=on
  MATLAB Function6 : MATLAB Function  TreatAsAtomicUnit=on
  MATLAB Function7 : MATLAB Function  Commented=on  TreatAsAtomicUnit=on
  MATLAB Function8 : MATLAB Function  Commented=on  TreatAsAtomicUnit=on
  MATLAB Function9 : MATLAB Function  Commented=on  TreatAsAtomicUnit=on
  Measured ZMP : sm_lib/Body Elements/Spherical Solid  Commented=on  GraphicAmbientColor=[0.15 0.15 0.15 1.0]  BasedOnType=Density  CenterOfMass=[0 0 0]  CenterOfMassUnits=m  GraphicDiffuseColor=[1.0 0.8 0.0]  Density=0.001  DensityUnits=kg/m^3  DoExposeReferenceFrame=on  GraphicEmissiveColor=[0.0 0.0 0.0 1.0]  ExportEntireGeometry=off  SerializedExposedGeometries=<ExposedGeometries/>  SerializedFrames=<Frames/>  MarkerShape=Sphere  MarkerSize=10  GraphicType=FromGeometry  InertiaType=CalculateFromGeometry  Mass=1  MassUnits=kg  MomentsOfInertia=[1 1 1]  MomentsOfInertiaUnits=kg*m^2  GraphicOpacity=1  ProductsOfInertia=[0 0 0]  ProductsOfInertiaUnits=kg*m^2  GraphicShininess=75  GraphicSpecularColor=[0.5 0.5 0.5 1.0]  SphereRadius=CoM_r  SphereRadiusUnits=mm  GraphicVisPropType=SimpleVisualProperties
  MechanismConfiguration : sm_lib/Utilities/Mechanism Configuration  UniformGravity=Constant  GravityVector=[0 0 -9.80665]  GravityVectorUnits=m/s^2  GravityUnits=m/s^2  LinearizationDelta=0.001  JointModeTransitionNonlinearIterations=2
  Mux{,2,8..9,14,23} (6 alike) : Mux  Inputs=3
  Mux1 : Mux  Inputs=5
  Mux{4..7,10..13,15..22} (16 alike) : Mux
  Mux3 : Mux  Inputs=5
  PS-Simulink Converter{,1..39,52..56} (45 alike) : nesl_utility/PS-Simulink Converter  PhysicalDomain=network_engine_domain  SubClassName=ps_output  LeftPortType=input  RightPortType=output  PseudoPeriodic=off  Frequencies=[]  Unit=inherit  AffineConversion=off
  PS-Simulink Converter{40..51} (12 alike) : nesl_utility/PS-Simulink Converter  Commented=on  PhysicalDomain=network_engine_domain  SubClassName=ps_output  LeftPortType=input  RightPortType=output  PseudoPeriodic=off  Frequencies=[]  Unit=inherit  AffineConversion=off
  Right Arm : Subsystem
  Right Leg : Subsystem
      settings: PortSchema="{\"entries\":[{\"content\":{\"sides\":[{\"content\":{\"connectorIds\":[]},\"type\":\"ConnectorPlacement.EquallySpacedRectSide\",\"uuid\":\"d191f65a-71ae-4d0f-881d-1faa5dc5cda7\"},{\"content\":{\"connectorIds\":[\"RConn1\",\"RConn2\",\"RConn3\",\"RConn4\"],\"side\":\"RIGHT\"},\"type\":\"ConnectorPlacement.EquallySpacedRectSide\",\"uuid\":\"ce1ac570-9f8e-4745-9f21-53e9bb963379\"},{\"content\":{\"connectorIds\":[],\"side\":\"TOP\"},\"type\":\"ConnectorPlacement.EquallySpacedRectSide\",\"uuid\":\"40ee9ab4-bf3a-46dc-9b28-4e0d14215192\"},{\"content\":{\"connectorIds\":[\"RConn5\"],\"side\":\"BOTTOM\"},\"type\":\"ConnectorPlacement.EquallySpacedRectSide\",\"uuid\":\"5fb5517d-9b38-409f-9583-f432a82d9ca6\"},{\"content\":{\"connectorIds\":[],\"side\":\"HIDDEN\"},\"type\":\"ConnectorPlacement.EquallySpacedRectSide\",\"uuid\":\"41464974-7d5c-490f-b26c-6f86a42437f7\"}]},\"type\":\"ConnectorPlacement.EquallySpacedConnector\",\"uuid\":\"8ec5d4ae-3ac0-497b-a9f7-427a802ecf00\"}],\"packageUris\":[\"http://schema.mathworks.com/mf0/Connector/R2020b\"],\"version\":\"1.0\"}"
  Right foot trajectory : Scope  NumInputPorts=3
  Simulink-PS Converter : nesl_utility/Simulink-PS Converter  Commented=on  PhysicalDomain=network_engine_domain  SubClassName=ps_input  LeftPortType=input  RightPortType=output  PseudoPeriodic=off  Frequencies=[]  NoiseDistribution=none  NoiseParameters=[]  Unit=mm  AffineConversion=off  FilteringAndDerivatives=filter  SimscapeFilterOrder=2  InputFilterTimeConstant=0.001  UdotUserProvided=0
  Simulink-PS Converter1 : nesl_utility/Simulink-PS Converter  Commented=on  PhysicalDomain=network_engine_domain  SubClassName=ps_input  LeftPortType=input  RightPortType=output  PseudoPeriodic=off  Frequencies=[]  NoiseDistribution=none  NoiseParameters=[]  Unit=mm  AffineConversion=off  FilteringAndDerivatives=filter  SimscapeFilterOrder=2  InputFilterTimeConstant=0.001  UdotUserProvided=0
  Simulink-PS Converter16 : nesl_utility/Simulink-PS Converter  PhysicalDomain=network_engine_domain  SubClassName=ps_input  LeftPortType=input  RightPortType=output  PseudoPeriodic=off  Frequencies=[]  NoiseDistribution=none  NoiseParameters=[]  Unit=mm  AffineConversion=off  FilteringAndDerivatives=filter  SimscapeFilterOrder=2  InputFilterTimeConstant=0.001  UdotUserProvided=0
  Simulink-PS Converter17 : nesl_utility/Simulink-PS Converter  PhysicalDomain=network_engine_domain  SubClassName=ps_input  LeftPortType=input  RightPortType=output  PseudoPeriodic=off  Frequencies=[]  NoiseDistribution=none  NoiseParameters=[]  Unit=mm  AffineConversion=off  FilteringAndDerivatives=filter  SimscapeFilterOrder=2  InputFilterTimeConstant=0.001  UdotUserProvided=0
  Simulink-PS Converter18 : nesl_utility/Simulink-PS Converter  PhysicalDomain=network_engine_domain  SubClassName=ps_input  LeftPortType=input  RightPortType=output  PseudoPeriodic=off  Frequencies=[]  NoiseDistribution=none  NoiseParameters=[]  Unit=mm  AffineConversion=off  FilteringAndDerivatives=filter  SimscapeFilterOrder=2  InputFilterTimeConstant=0.001  UdotUserProvided=0
  Simulink-PS Converter2 : nesl_utility/Simulink-PS Converter  Commented=on  PhysicalDomain=network_engine_domain  SubClassName=ps_input  LeftPortType=input  RightPortType=output  PseudoPeriodic=off  Frequencies=[]  NoiseDistribution=none  NoiseParameters=[]  Unit=mm  AffineConversion=off  FilteringAndDerivatives=filter  SimscapeFilterOrder=2  InputFilterTimeConstant=0.001  UdotUserProvided=0
  Solver Configuration : nesl_utility/Solver Configuration  PhysicalDomain=network_engine_domain  SubClassName=solver  LeftPortType=input  RightPortType=generic  Tones=[]  Harmonics=[]  SimulateNoise=off  Profile=off  UseLocalSampling=off  EnableSwitchedLinearOptims=on  FrequencyDomain=off  UseCCode=off  RelTol=0.001  AbsTol=1e-06  MinStep=1e-09  ToWorkspace=off  RevertToSquareIcSolve=off  NumHomotopyIterations=100  PhasorMode=off  PhasorModeNumHarmonics=1  DoDC=off  ResidualTolerance=1e-9  UseLocalSolver=off  LocalSolverChoice=NE_BACKWARD_EULER_ADVANCER  LocalSolverSampleTime=0.001  DoFixedCost=off  MaxNonlinIter=3  MaxModeIter=2  ComputeImpulses=off  ImpulseIterations=2  LinearAlgebra=auto  EquationFormulation=NE_TIME_EF  DelaysMemoryBudget=5096  AutomaticFiltering=on  FilteringTimeConstant=0.001  PartitionStorageMethod=AS_NEEDED  PartitionMemoryBudget=1024  PartitionMethod=ROBUST
  Spatial Contact Force{,1..7} (8 alike) : sm_lib/Forces and Torques/Spatial Contact Force  CoefficientOfDynamicFriction=Coff_dyn  CoefficientOfStaticFriction=Coff_static  NormalDamping=Contact_Damping  NormalDampingUnits=N/(m/s)  NormalStiffness=Contact_Stiff  NormalStiffnessUnits=N/m  FrictionalCriticalVelocity=V_critical  FrictionalCriticalVelocityUnits=m/s  ZeroCrossDetectContactStartAndEnd=off  SenseFrictionalForceMagnitude=on  SenseNormalForceMagnitude=on  SenseSeparationDistance=off  NormalTransitionRegionWidth=Contact_Trans  NormalTransitionRegionWidthUnits=m  FrictionType=SmoothStickSlip
  Spherical Solid{,1..7} (8 alike) : sm_lib/Body Elements/Spherical Solid  GraphicAmbientColor=[0.15 0.15 0.15 1.0]  BasedOnType=Density  CenterOfMass=[0 0 0]  CenterOfMassUnits=m  GraphicDiffuseColor=Contact_color  Density=0.0001  DensityUnits=kg/m^3  DoExposeReferenceFrame=on  GraphicEmissiveColor=[0.0 0.0 0.0 1.0]  ExportEntireGeometry=on  SerializedExposedGeometries=<ExposedGeometries><ExposedGeometry><RawGeometryId>entire</RawGeometryId><ExposedGeometryId>G</ExposedGeometryId></ExposedGeometry></ExposedGeometries>  SerializedFrames=<Frames/>  MarkerShape=Sphere  MarkerSize=10  GraphicType=FromGeometry  InertiaType=CalculateFromGeometry  Mass=1  MassUnits=kg  MomentsOfInertia=[1 1 1]  MomentsOfInertiaUnits=kg*m^2  GraphicOpacity=1.0  ProductsOfInertia=[0 0 0]  ProductsOfInertiaUnits=kg*m^2  GraphicShininess=75  GraphicSpecularColor=[0.5 0.5 0.5 1.0]  SphereRadius=Contact_r  SphereRadiusUnits=mm  GraphicVisPropType=SimpleVisualProperties
  Step time : Constant  Value=0.5
  To Workspace : ToWorkspace  Commented=on  VariableName=calc_slip_x  SaveFormat=Timeseries  SampleTime=-1
  To Workspace1 : ToWorkspace  Commented=on  VariableName=calc_slip_y  SaveFormat=Timeseries  SampleTime=-1
  To Workspace10 : ToWorkspace  VariableName=left_friction  SaveFormat=Timeseries  SampleTime=-1
  To Workspace11 : ToWorkspace  VariableName=right_friction  SaveFormat=Timeseries  SampleTime=-1
  To Workspace12 : ToWorkspace  VariableName=Left_Vel_X  SaveFormat=Timeseries  SampleTime=-1
  To Workspace13 : ToWorkspace  VariableName=Left_Vel_Y  SaveFormat=Timeseries  SampleTime=-1
  To Workspace14 : ToWorkspace  VariableName=Right_Vel_X  SaveFormat=Timeseries  SampleTime=-1
  To Workspace15 : ToWorkspace  VariableName=Right_Vel_Y  SaveFormat=Timeseries  SampleTime=-1
  To Workspace16 : ToWorkspace  VariableName=Left_Slip  SaveFormat=Timeseries  SampleTime=-1
  To Workspace17 : ToWorkspace  Commented=on  VariableName=mag_calculated  SaveFormat=Timeseries  SampleTime=-1
  To Workspace18 : ToWorkspace  Commented=on  VariableName=accel  SaveFormat=Timeseries  SampleTime=-1
  To Workspace19 : ToWorkspace  VariableName=Right_Slip  SaveFormat=Timeseries  SampleTime=-1
  To Workspace2 : ToWorkspace  Commented=on  VariableName=zmp_x  SaveFormat=Timeseries  SampleTime=-1
  To Workspace20 : ToWorkspace  VariableName=com_accel_ang  SaveFormat=Timeseries  SampleTime=-1
  To Workspace21 : ToWorkspace  VariableName=force_com  SaveFormat=Timeseries  SampleTime=-1
  To Workspace22 : ToWorkspace  VariableName=torque_com  SaveFormat=Timeseries  SampleTime=-1
  To Workspace3 : ToWorkspace  Commented=on  VariableName=zmp_y  SaveFormat=Timeseries  SampleTime=-1
  To Workspace4 : ToWorkspace  VariableName=left_force  SaveFormat=Timeseries  SampleTime=-1
  To Workspace5 : ToWorkspace  VariableName=right_force  SaveFormat=Timeseries  SampleTime=-1
  To Workspace6 : ToWorkspace  Commented=on  VariableName=inertial_force_x  SaveFormat=Timeseries  SampleTime=-1
  To Workspace7 : ToWorkspace  Commented=on  VariableName=inertial_force_y  SaveFormat=Timeseries  SampleTime=-1
  To Workspace8 : ToWorkspace  Commented=on  VariableName=reaction_force_x  SaveFormat=Timeseries  SampleTime=-1
  To Workspace9 : ToWorkspace  Commented=on  VariableName=reaction_force_y  SaveFormat=Timeseries  SampleTime=-1
  Transform Sensor{,1..7} (8 alike) : sm_lib/Frames and Transforms/Transform Sensor  MeasurementFrame=Base  SenseAngle=off  SenseAxis=off  SenseAngle1=off  SenseAngle2=off  SenseAngle3=off  SenseQ=off  SenseR=off  SenseOmegaX=off  SenseOmegaY=off  SenseOmegaZ=off  SenseOmega1=off  SenseOmega2=off  SenseOmega3=off  SenseQDot=off  SenseRDot=off  SenseAlphaX=off  SenseAlphaY=off  SenseAlphaZ=off  SenseAlpha1=off  SenseAlpha2=off  SenseAlpha3=off  SenseQDDot=off  SenseRDDot=off  SenseX=on  SenseY=on  SenseZ=on  SenseRad=off  SenseAzim=off  SenseDist=off  SenseInc=off  SenseXDot=off  SenseYDot=off  SenseZDot=off  SenseRadDot=off  SenseAzimDot=off  SenseDistDot=off  SenseIncDot=off  SenseXDDot=off  SenseYDDot=off  SenseZDDot=off  SenseRadDDot=off  SenseAzimDDot=off  SenseDistDDot=off  SenseIncDDot=off
  Transform Sensor{10,13..15} (4 alike) : sm_lib/Frames and Transforms/Transform Sensor  MeasurementFrame=Base  SenseAngle=off  SenseAxis=off  SenseAngle1=off  SenseAngle2=off  SenseAngle3=off  SenseQ=off  SenseR=off  SenseOmegaX=off  SenseOmegaY=off  SenseOmegaZ=off  SenseOmega1=off  SenseOmega2=off  SenseOmega3=off  SenseQDot=off  SenseRDot=off  SenseAlphaX=off  SenseAlphaY=off  SenseAlphaZ=off  SenseAlpha1=off  SenseAlpha2=off  SenseAlpha3=off  SenseQDDot=off  SenseRDDot=off  SenseX=off  SenseY=off  SenseZ=off  SenseRad=off  SenseAzim=off  SenseDist=off  SenseInc=off  SenseXDot=on  SenseYDot=on  SenseZDot=off  SenseRadDot=off  SenseAzimDot=off  SenseDistDot=off  SenseIncDot=off  SenseXDDot=off  SenseYDDot=off  SenseZDDot=off  SenseRadDDot=off  SenseAzimDDot=off  SenseDistDDot=off  SenseIncDDot=off
  Transform Sensor{8..9,11..12} (4 alike) : sm_lib/Frames and Transforms/Transform Sensor  MeasurementFrame=World  SenseAngle=off  SenseAxis=off  SenseAngle1=off  SenseAngle2=off  SenseAngle3=off  SenseQ=off  SenseR=off  SenseOmegaX=off  SenseOmegaY=off  SenseOmegaZ=off  SenseOmega1=off  SenseOmega2=off  SenseOmega3=off  SenseQDot=off  SenseRDot=off  SenseAlphaX=off  SenseAlphaY=off  SenseAlphaZ=off  SenseAlpha1=off  SenseAlpha2=off  SenseAlpha3=off  SenseQDDot=off  SenseRDDot=off  SenseX=off  SenseY=off  SenseZ=off  SenseRad=off  SenseAzim=off  SenseDist=off  SenseInc=off  SenseXDot=on  SenseYDot=on  SenseZDot=off  SenseRadDot=off  SenseAzimDot=off  SenseDistDot=off  SenseIncDot=off  SenseXDDot=off  SenseYDDot=off  SenseZDDot=off  SenseRadDDot=off  SenseAzimDDot=off  SenseDistDDot=off  SenseIncDDot=off
  Transform1 : sm_lib/Frames and Transforms/Rigid Transform  TranslationMethod=StandardAxis  TranslationStandardOffset=194.5  TranslationLengthUnit=mm  TranslationStandardAxis=-Z  TranslationCartesianOffset=smiData.RigidTransform(2).translation-[0, 0, -169]  TranslationROffset=0  TranslationROffsetUnits=m  TranslationZOffset=0  TranslationZOffsetUnits=m  TranslationThetaOffset=0  TranslationThetaOffsetUnits=deg  RotationMethod=None  RotationAngleUnits=rad  RotationStandardAxis=+Z  RotationAngle=smiData.RigidTransform(2).angle  RotationArbitraryAxis=smiData.RigidTransform(2).axis  FollAlignAxisA=+X  BaseAlignAxisA=+Y  FollAlignAxisB=+Y  BaseAlignAxisB=+Z  RotationSequenceAxes=FollowerAxes  RotationSequence=XYX  RotationSequenceAngles=[0 0 0]  RotationSequenceAnglesUnits=deg  RotationMatrix=[1 0 0; 0 1 0; 0 0 1]
  Unit Delay : UnitDelay  InitialCondition=pi/3  SampleTime=-1  HasFrameUpgradeWarning=on
  Unit Delay1 : UnitDelay  InitialCondition=-pi/3  SampleTime=-1  HasFrameUpgradeWarning=on
  Unit Delay2 : UnitDelay  SampleTime=-1  HasFrameUpgradeWarning=on
  Unit Delay3 : UnitDelay  SampleTime=-1  HasFrameUpgradeWarning=on
  World : sm_lib/Frames and Transforms/World Frame
  Zmp Location2 : sm_lib/Body Elements/Spherical Solid  Commented=on  GraphicAmbientColor=[0.15 0.15 0.15 1.0]  BasedOnType=Density  CenterOfMass=[0 0 0]  CenterOfMassUnits=m  GraphicDiffuseColor=ZMP2_color  Density=0.00001  DensityUnits=kg/m^3  DoExposeReferenceFrame=on  GraphicEmissiveColor=[0.0 0.0 0.0 1.0]  ExportEntireGeometry=off  SerializedExposedGeometries=<ExposedGeometries/>  SerializedFrames=<Frames/>  MarkerShape=Sphere  MarkerSize=10  GraphicType=FromGeometry  InertiaType=CalculateFromGeometry  Mass=1  MassUnits=kg  MomentsOfInertia=[1 1 1]  MomentsOfInertiaUnits=kg*m^2  GraphicOpacity=1  ProductsOfInertia=[0 0 0]  ProductsOfInertiaUnits=kg*m^2  GraphicShininess=75  GraphicSpecularColor=[0.5 0.5 0.5 1.0]  SphereRadius=5  SphereRadiusUnits=mm  GraphicVisPropType=SimpleVisualProperties
  pirch_LF : Constant  Value=0
  pitch_RF : Constant  Value=0
  roll_LF : Constant  Value=0
  roll_RF : Constant  Value=0
  x_LH : Constant  Value=0
  x_RH : Constant  Value=0
  y_LH : Constant  Value=174-100
  y_RH : Constant  Value=-174+100
  z_LH : Constant  Value=-12-110
  z_RH : Constant  Value=-110-12
  XY Graph : simulink/Sinks/XY Graph  IOType=viewer  xmin=-1  xmax=1  ymin=-1  ymax=1  st=-1
  tag scope: LF_angle=global, LH_angle=global, RF_angle=global, RH_angle=global, joint_angle=global, joint_vel=global
  wires:
  x_RH/1 -> MATLAB Function1/1(x_RH_in)
  pitch_RF/1 -> MATLAB Function3/5(pitch_RF)
  roll_RF/1 -> MATLAB Function3/4(roll_RF)
  y_LH/1 -> MATLAB Function2/2(y_LH_in)
  x_LH/1 -> MATLAB Function2/1(x_LH_in)
  roll_LF/1 -> MATLAB Function/4(roll_LF)
  pirch_LF/1 -> MATLAB Function/5(pitch_LF)
  MATLAB Function1/1(th1) -> Mux/1
  MATLAB Function2/3(th6) -> Mux2/3
  MATLAB Function3/1(th7) -> Mux1/1
  MATLAB Function3/3(th11) -> Mux1/3
  MATLAB Function3/4(th13) -> Mux1/4
  MATLAB Function3/5(th15) -> Mux1/5
  MATLAB Function/1(th8) -> Mux3/1
  MATLAB Function/2(th10) -> Mux3/2
  MATLAB Function/3(th12) -> Mux3/3
  MATLAB Function/4(th14) -> Mux3/4
  z_RH/1 -> MATLAB Function1/3(z_RH_in)
  y_RH/1 -> MATLAB Function1/2(y_RH_in)
  z_LH/1 -> MATLAB Function2/3(z_LH_in)
  MATLAB Function2/1(th2) -> Mux2/1
  MATLAB Function3/2(th9) -> Mux1/2
  MATLAB Function/5(th16) -> Mux3/5
  MATLAB Function1/3(th5) -> Mux/3
  "Clock "/1 -> MATLAB Function6/1(time)
  Mux/1 -> [RH_angle]
  Mux1/1 -> [RF_angle]
  Mux3/1 -> [LF_angle]
  Mux2/1 -> [LH_angle]
  [RH_angle] -> Mux4/1
  [LH_angle] -> Mux4/2
  [RF_angle] -> Mux4/3
  [LF_angle] -> Mux4/4
  Mux4/1 -> [joint_angle]
  Mux7/1 -> [joint_vel]
  [RH_vel] -> Mux7/1
  [LH_vel] -> Mux7/2
  [RF_vel] -> Mux7/3
  [LH_vel] -> Mux7/4
  MATLAB Function6/1(x_RF) -> Right foot trajectory/1, Mux8/1
  MATLAB Function6/2(y_RF) -> Right foot trajectory/2, Mux8/2
  MATLAB Function6/3(z_RF) -> Right foot trajectory/3, Mux8/3
  Mux8/1 -> [pos_RF]
  MATLAB Function6/5(y_LF) -> Mux9/2, Left foot trajectory/2
  MATLAB Function6/6(z_LF) -> Left foot trajectory/3, Mux9/3
  MATLAB Function6/4(x_LF) -> Left foot trajectory/1, Mux9/1
  Mux9/1 -> [pos_LF]
  [pos_LF] -> Demux5/1
  "Foot Lift timing Constant (0~1) if 0, feet are not lifted"/1 -> MATLAB Function6/2(tau)
  Step time/1 -> MATLAB Function6/3(step_time)
  [pos_RF] -> Demux4/1
  Demux/2 -> Simulink-PS Converter17/1
  Demux/1 -> Simulink-PS Converter16/1
  Demux/3 -> Simulink-PS Converter18/1
  [joint_angle] -> MATLAB Function4/1(joint_angle)
  MATLAB Function4/1(P_CoM_wholebody) -> [CoM], Demux/1
  Low-pass filter_L Force Sensors/1(f1) -> Mux5/1
  Low-pass filter_L Force Sensors/2(f2) -> Mux5/2
  Low-pass filter_L Force Sensors/3(f3) -> Mux5/3
  Low-pass filter_L Force Sensors/4(f4) -> Mux5/4
  Mux5/1 -> [Left_Force_Sensors]
  Low-pass filter_R Force Sensors/1(f1) -> Mux6/1
  Low-pass filter_R Force Sensors/2(f2) -> Mux6/2
  Low-pass filter_R Force Sensors/3(f3) -> Mux6/3
  Low-pass filter_R Force Sensors/4(f4) -> Mux6/4
  Mux6/1 -> [Right_Force_Sensors]
  Mux10/1 -> [L_Force_Sensors_PosX]
  Mux11/1 -> [L_Force_Sensors_PosY]
  PS-Simulink Converter/1 -> Mux10/1
  PS-Simulink Converter1/1 -> Mux10/2
  PS-Simulink Converter2/1 -> Mux10/3
  PS-Simulink Converter3/1 -> Mux10/4
  PS-Simulink Converter4/1 -> Mux11/1
  PS-Simulink Converter5/1 -> Mux11/2
  PS-Simulink Converter6/1 -> Mux11/3
  PS-Simulink Converter7/1 -> Mux11/4
  PS-Simulink Converter15/1 -> Mux13/4
  PS-Simulink Converter12/1 -> Mux13/1
  PS-Simulink Converter14/1 -> Mux13/3
  PS-Simulink Converter9/1 -> Mux12/2
  PS-Simulink Converter13/1 -> Mux13/2
  Mux12/1 -> [R_Force_Sensors_PosX]
  PS-Simulink Converter10/1 -> Mux12/3
  PS-Simulink Converter11/1 -> Mux12/4
  PS-Simulink Converter8/1 -> Mux12/1
  Mux13/1 -> [R_Force_Sensors_PosY]
  From4/1 -> MATLAB Function8/3(l_x)
  From7/1 -> MATLAB Function8/4(l_y)
  From11/1 -> MATLAB Function8/1(Left_Force_Sensors)
  From16/1 -> MATLAB Function8/6(r_y)
  From15/1 -> MATLAB Function8/5(r_x)
  From12/1 -> MATLAB Function8/2(Right_Force_Sensors)
  Constant/1 -> Simulink-PS Converter2/1
  From17/1 -> MATLAB Function11/1(CoM), MATLAB Function10/1(CoM), MATLAB Function9/3(CoM)
  Low-pass filter Accel Sensor/1(ax) -> Mux14/1
  Low-pass filter Accel Sensor/2(ay) -> Mux14/2
  Low-pass filter Accel Sensor/3(az) -> Mux14/3
  Mux14/1 -> [CoM_Accel]
  From18/1 -> To Workspace18/1, MATLAB Function10/2(a)
  MATLAB Function10/1(p_x) -> MATLAB Function9/1(p_x)
  MATLAB Function10/2(p_y) -> MATLAB Function9/2(p_y)
  Mux16/1 -> [R_Force_Sensors_Friction]
  Mux15/1 -> [L_Force_Sensors_Friction]
  MATLAB Function9/1(force_x) -> To Workspace6/1, MATLAB Function12/1(inertial_x)
  MATLAB Function9/2(force_y) -> To Workspace7/1, MATLAB Function12/2(inertial_y)
  MATLAB Function11/1(reaction_x) -> To Workspace8/1, MATLAB Function12/3(reaction_x)
  MATLAB Function11/2(reaction_y) -> MATLAB Function12/4(reaction_y), To Workspace9/1
  [Left_Force_Sensors] -> To Workspace4/1
  [Right_Force_Sensors] -> To Workspace5/1
  MATLAB Function8/1(p_x) -> Simulink-PS Converter/1
  MATLAB Function8/2(p_y) -> Simulink-PS Converter1/1
  MATLAB Function12/1(slip_x) -> To Workspace/1
  MATLAB Function12/2(slip_y) -> To Workspace1/1
  [R_Force_Sensors_Friction] -> To Workspace11/1
  [L_Force_Sensors_Friction] -> To Workspace10/1
  [L_Force_Sensors_Vx] -> To Workspace12/1
  [L_Force_Sensors_Vy] -> To Workspace13/1
  [R_Force_Sensors_Vy] -> To Workspace15/1
  [R_Force_Sensors_Vx] -> To Workspace14/1
  Mux18/1 -> [L_Force_Sensors_Vy]
  Mux17/1 -> [L_Force_Sensors_Vx]
  Mux20/1 -> [R_Force_Sensors_Vy]
  Mux19/1 -> [R_Force_Sensors_Vx]
  PS-Simulink Converter19/1 -> Mux19/1
  PS-Simulink Converter24/1 -> Mux19/2
  PS-Simulink Converter25/1 -> Mux19/3
  PS-Simulink Converter27/1 -> Mux19/4
  PS-Simulink Converter26/1 -> Mux20/1
  PS-Simulink Converter16/1 -> Mux20/2
  PS-Simulink Converter17/1 -> Mux20/3
  PS-Simulink Converter18/1 -> Mux20/4
  PS-Simulink Converter22/1 -> Mux18/4
  PS-Simulink Converter21/1 -> Mux18/3
  PS-Simulink Converter20/1 -> Mux18/2
  PS-Simulink Converter35/1 -> Mux18/1
  PS-Simulink Converter32/1 -> Mux17/1
  PS-Simulink Converter33/1 -> Mux17/2
  PS-Simulink Converter34/1 -> Mux17/3
  PS-Simulink Converter36/1 -> Mux17/4
  [L_Force_Sensors_Vy] -> MATLAB Function5/5(L_vx)
  [L_Force_Sensors_Vx] -> MATLAB Function5/6(L_vy)
  [R_Force_Sensors_Vy] -> MATLAB Function5/7(R_vx)
  [R_Force_Sensors_Vx] -> MATLAB Function5/8(R_vy)
  [R_Force_Sensors_Friction] -> MATLAB Function5/3(Right_Friction_Sensor)
  [L_Force_Sensors_Friction] -> MATLAB Function5/1(Left_Friction_Sensor)
  [Left_Force_Sensors] -> MATLAB Function5/2(Left_Normal_Force)
  [Right_Force_Sensors] -> MATLAB Function5/4(Right_Normal_Force)
  MATLAB Function5/1(Left_Slip) -> To Workspace16/1
  MATLAB Function5/2(Right_Slip) -> To Workspace19/1
  Demux5/1 -> MATLAB Function/1(x_LF_in)
  Demux5/3 -> MATLAB Function/3(z_LF_in)
  Demux4/1 -> MATLAB Function3/1(x_RF_in)
  Demux4/2 -> MATLAB Function3/2(y_RF_in)
  Demux4/3 -> MATLAB Function3/3(z_RF_in)
  Low-pass filter_L Force Sensors1/1(f1) -> Mux15/1
  Low-pass filter_L Force Sensors1/2(f2) -> Mux15/2
  Low-pass filter_L Force Sensors1/3(f3) -> Mux15/3
  Low-pass filter_L Force Sensors1/4(f4) -> Mux15/4
  Low-pass filter_L Force Sensors2/1(f1) -> Mux16/1
  Low-pass filter_L Force Sensors2/2(f2) -> Mux16/2
  Low-pass filter_L Force Sensors2/3(f3) -> Mux16/3
  Low-pass filter_L Force Sensors2/4(f4) -> Mux16/4
  From30/1 -> MATLAB Function11/5(Right_Friction_Sensors)
  From29/1 -> MATLAB Function11/4(Left_Friction_Sensors)
  From31/1 -> MATLAB Function11/6(L_x)
  From32/1 -> MATLAB Function11/7(L_y)
  From33/1 -> MATLAB Function11/9(R_x)
  From34/1 -> MATLAB Function11/10(R_y)
  From41/1 -> MATLAB Function11/2(Left_Normal_Force)
  From42/1 -> MATLAB Function11/3(Right_Normal_Force)
  Mux21/1 -> [L_Force_Sensors_PosZ]
  PS-Simulink Converter37/1 -> Mux21/1
  PS-Simulink Converter31/1 -> Mux21/2
  PS-Simulink Converter38/1 -> Mux21/3
  PS-Simulink Converter30/1 -> Mux21/4
  PS-Simulink Converter52/1 -> Mux22/2
  PS-Simulink Converter54/1 -> Mux22/4
  PS-Simulink Converter53/1 -> Mux22/3
  Mux22/1 -> [R_Force_Sensors_PosZ]
  PS-Simulink Converter55/1 -> Mux22/1
  From43/1 -> MATLAB Function11/11(R_z)
  From44/1 -> MATLAB Function11/8(L_z)
  Demux5/2 -> MATLAB Function/2(y_LF_in)
  Mux23/1 -> To Workspace20/1
  PS-Simulink Converter28/1 -> Mux23/2
  PS-Simulink Converter23/1 -> Mux23/1
  PS-Simulink Converter29/1 -> Mux23/3
  PS-Simulink Converter39/1 -> To Workspace21/1
  PS-Simulink Converter56/1 -> To Workspace22/1
  Unit Delay2/1 -> MATLAB Function13/4(R_v)
  Unit Delay3/1 -> MATLAB Function13/3(L_v)
  [Right_Force_Sensors] -> MATLAB Function13/2(Right_Normal_Force)
  [Left_Force_Sensors] -> MATLAB Function13/1(Left_Normal_Force)
  Unit Delay/1 -> MATLAB Function13/5(L_p)
  Unit Delay1/1 -> MATLAB Function13/6(R_p)
  MATLAB Function13/3(angle_right_arm) -> Unit Delay1/1, [Right_Arm_3]
  MATLAB Function13/4(angle_left_arm) -> Unit Delay/1, [Left_Arm_4]
  [Left_Arm_4] -> Mux2/2
  [Right_Arm_3] -> Mux/2
  MATLAB Function13/2(v_left_arm) -> Unit Delay3/1
  MATLAB Function13/1(v_right_arm) -> Unit Delay2/1
  connections:
  Transform1/RConn1 -- Floor/RConn1
  Floor/LConn1 -- Spatial Contact Force1/LConn1 -- Spatial Contact Force6/LConn1 -- Spatial Contact Force7/LConn1 -- Spatial Contact Force5/LConn1 -- Spatial Contact Force/LConn1 -- Spatial Contact Force4/LConn1 -- Spatial Contact Force3/LConn1 -- Spatial Contact Force2/LConn1
  Spatial Contact Force/RConn1 -- Spherical Solid/LConn1
  Spherical Solid3/LConn1 -- Spatial Contact Force3/RConn1
  Spherical Solid2/LConn1 -- Spatial Contact Force4/RConn1
  Spherical Solid1/LConn1 -- Spatial Contact Force2/RConn1
  Spherical Solid7/LConn1 -- Spatial Contact Force6/RConn1
  Spherical Solid4/LConn1 -- Spatial Contact Force5/RConn1
  Spherical Solid5/LConn1 -- Spatial Contact Force1/RConn1
  Spherical Solid6/LConn1 -- Spatial Contact Force7/RConn1
  Body_1_RIGID/LConn1 -- Right Arm/RConn1
  Body_1_RIGID/RConn1 -- Left Arm/LConn1
  Body_1_RIGID/RConn2 -- Right Leg/RConn5
  Spherical Solid1/RConn1 -- Transform Sensor1/RConn1 -- Transform Sensor9/RConn1 -- Right Leg/RConn2
  Body_1_RIGID/RConn3 -- Left Leg/LConn1
  Spherical Solid5/RConn1 -- Transform Sensor10/RConn1 -- Transform Sensor4/RConn1 -- Left Leg/RConn1
  Spherical Solid4/RConn1 -- Transform Sensor5/RConn1 -- Transform Sensor13/RConn1 -- Left Leg/RConn2
  Spherical Solid7/RConn1 -- Transform Sensor14/RConn1 -- Transform Sensor6/RConn1 -- Left Leg/RConn3
  Spherical Solid6/RConn1 -- Left Leg/RConn4 -- Transform Sensor15/RConn1 -- Transform Sensor7/RConn1
  MechanismConfiguration/RConn1 -- World/RConn1 -- 6-DOF Joint/RConn1 -- Transform1/LConn1 -- Solver Configuration/RConn1
  Spatial Contact Force/RConn2 -- Low-pass filter_R Force Sensors/LConn1
  Spatial Contact Force2/RConn2 -- Low-pass filter_R Force Sensors/LConn2
  Spatial Contact Force4/RConn2 -- Low-pass filter_R Force Sensors/LConn3
  Spatial Contact Force3/RConn2 -- Low-pass filter_R Force Sensors/LConn4
  Low-pass filter_L Force Sensors/LConn1 -- Spatial Contact Force1/RConn2
  Low-pass filter_L Force Sensors/LConn2 -- Spatial Contact Force5/RConn2
  Low-pass filter_L Force Sensors/LConn3 -- Spatial Contact Force6/RConn2
  Low-pass filter_L Force Sensors/LConn4 -- Spatial Contact Force7/RConn2
  Spherical Solid3/RConn1 -- Transform Sensor3/RConn1 -- Transform Sensor12/RConn1 -- Right Leg/RConn4
  Right Leg/RConn1 -- Transform Sensor/RConn1 -- Transform Sensor8/RConn1 -- Spherical Solid/RConn1
  Spherical Solid2/RConn1 -- Transform Sensor2/RConn1 -- Transform Sensor11/RConn1 -- Right Leg/RConn3
  Simulink-PS Converter16/RConn1 -- 6-DOF Joint1/LConn2
  Simulink-PS Converter17/RConn1 -- 6-DOF Joint1/LConn3
  Simulink-PS Converter18/RConn1 -- 6-DOF Joint1/LConn4
  CoM Location/RConn1 -- Accel Sensor/RConn1 -- 6-DOF Joint1/RConn1
  Body_1_RIGID/LConn2 -- 6-DOF Joint2/LConn1 -- 6-DOF Joint1/LConn1 -- Transform Sensor9/LConn1 -- Transform Sensor8/LConn1 -- Transform Sensor3/LConn1 -- Transform Sensor2/LConn1 -- Transform Sensor1/LConn1 -- Transform Sensor/LConn1 -- Transform Sensor15/LConn1 -- Transform Sensor14/LConn1 -- Transform Sensor13/LConn1 -- Transform Sensor10/LConn1 -- Transform Sensor7/LConn1 -- Transform Sensor6/LConn1 -- Transform Sensor5/LConn1 -- Transform Sensor4/LConn1 -- 6-DOF Joint/LConn1
  Transform Sensor/RConn2 -- PS-Simulink Converter8/LConn1
  Transform Sensor1/RConn2 -- PS-Simulink Converter9/LConn1
  Transform Sensor2/RConn2 -- PS-Simulink Converter10/LConn1
  Transform Sensor3/RConn2 -- PS-Simulink Converter11/LConn1
  Transform Sensor/RConn3 -- PS-Simulink Converter12/LConn1
  Transform Sensor1/RConn3 -- PS-Simulink Converter13/LConn1
  Transform Sensor2/RConn3 -- PS-Simulink Converter14/LConn1
  Transform Sensor3/RConn3 -- PS-Simulink Converter15/LConn1
  Transform Sensor4/RConn2 -- PS-Simulink Converter/LConn1
  Transform Sensor5/RConn2 -- PS-Simulink Converter1/LConn1
  Transform Sensor6/RConn2 -- PS-Simulink Converter2/LConn1
  Transform Sensor7/RConn2 -- PS-Simulink Converter3/LConn1
  Transform Sensor5/RConn3 -- PS-Simulink Converter5/LConn1
  Transform Sensor6/RConn3 -- PS-Simulink Converter6/LConn1
  Transform Sensor7/RConn3 -- PS-Simulink Converter7/LConn1
  Simulink-PS Converter/RConn1 -- 6-DOF Joint2/LConn2
  Simulink-PS Converter1/RConn1 -- 6-DOF Joint2/LConn3
  Simulink-PS Converter2/RConn1 -- 6-DOF Joint2/LConn4
  Measured ZMP/RConn1 -- 6-DOF Joint2/RConn1
  Spatial Contact Force1/RConn3 -- Low-pass filter_L Force Sensors1/LConn1
  Spatial Contact Force5/RConn3 -- Low-pass filter_L Force Sensors1/LConn2
  Low-pass filter_L Force Sensors1/LConn3 -- Spatial Contact Force6/RConn3
  Spatial Contact Force7/RConn3 -- Low-pass filter_L Force Sensors1/LConn4
  Low-pass filter_L Force Sensors2/LConn1 -- Spatial Contact Force/RConn3
  Spatial Contact Force2/RConn3 -- Low-pass filter_L Force Sensors2/LConn2
  Spatial Contact Force4/RConn3 -- Low-pass filter_L Force Sensors2/LConn3
  Spatial Contact Force3/RConn3 -- Low-pass filter_L Force Sensors2/LConn4
  PS-Simulink Converter4/LConn1 -- Transform Sensor4/RConn3
  PS-Simulink Converter19/LConn1 -- Transform Sensor8/RConn2
  PS-Simulink Converter24/LConn1 -- Transform Sensor9/RConn2
  PS-Simulink Converter25/LConn1 -- Transform Sensor11/RConn2
  Transform Sensor12/RConn2 -- PS-Simulink Converter27/LConn1
  Transform Sensor8/RConn3 -- PS-Simulink Converter26/LConn1
  Transform Sensor9/RConn3 -- PS-Simulink Converter16/LConn1
  Transform Sensor11/RConn3 -- PS-Simulink Converter17/LConn1
  Transform Sensor12/RConn3 -- PS-Simulink Converter18/LConn1
  Transform Sensor10/RConn2 -- PS-Simulink Converter32/LConn1
  Transform Sensor13/RConn2 -- PS-Simulink Converter33/LConn1
  Transform Sensor14/RConn2 -- PS-Simulink Converter34/LConn1
  Transform Sensor15/RConn2 -- PS-Simulink Converter36/LConn1
  Transform Sensor10/RConn3 -- PS-Simulink Converter35/LConn1
  Transform Sensor13/RConn3 -- PS-Simulink Converter20/LConn1
  PS-Simulink Converter21/LConn1 -- Transform Sensor14/RConn3
  Transform Sensor15/RConn3 -- PS-Simulink Converter22/LConn1
  Transform Sensor7/RConn4 -- PS-Simulink Converter30/LConn1
  Transform Sensor6/RConn4 -- PS-Simulink Converter38/LConn1
  Transform Sensor5/RConn4 -- PS-Simulink Converter31/LConn1
  Transform Sensor4/RConn4 -- PS-Simulink Converter37/LConn1
  Transform Sensor/RConn4 -- PS-Simulink Converter55/LConn1
  Transform Sensor1/RConn4 -- PS-Simulink Converter52/LConn1
  Transform Sensor2/RConn4 -- PS-Simulink Converter53/LConn1
  Transform Sensor3/RConn4 -- PS-Simulink Converter54/LConn1
  Low-pass filter Accel Sensor/LConn1 -- Accel Sensor/RConn5
  Low-pass filter Accel Sensor/LConn2 -- Accel Sensor/RConn6
  Low-pass filter Accel Sensor/LConn3 -- Accel Sensor/RConn7
  PS-Simulink Converter23/LConn1 -- Accel Sensor/RConn2
  PS-Simulink Converter28/LConn1 -- Accel Sensor/RConn3
  PS-Simulink Converter29/LConn1 -- Accel Sensor/RConn4
  6-DOF Joint1/RConn2 -- PS-Simulink Converter39/LConn1
  PS-Simulink Converter56/LConn1 -- 6-DOF Joint1/RConn3
